simulink model "metux_controller"  (R2025b)
settings: Solver=FixedStepDiscrete  StartTime=0.0  StopTime=10  FixedStep=1/1000  RelTol=1e-3
InitFcn:
  | motor_parameters;
  | plant_parameters;
  | %load("dropLookup.mat");
  | %load("force_function.mat");
model workspace (MAT data in the model file):
  stepGain = 60
values from neighbouring files (symbols this model uses):
  enableKalmanForPositionEst = 1    [motor_parameters.m]
  enableKalmanForVelocityEst = 1    [motor_parameters.m]
  position_controller_Ts = 1e-3    (= 0.001)    [motor_parameters.m]
  velocity_controller_Ts = 1e-3    (= 0.001)    [motor_parameters.m]
libraries: subsystems x4
settings Model: TunableVars=enableKalmanForPositionEst,enableKalmanForVelocityEst,position_controller,velocity_controller,lidar_height,kalkis_target_height,Nozzle,Cmdot,attitude_controller,hwil  TunableVarsStorageClass=ExportedGlobal,ExportedGlobal,ExportedGlobal,ExportedGlobal,Auto,Auto,Auto,Auto,Auto,Auto  TunableVarsTypeQualifier=,,,,,,,,,  Creator=karadeli  LastModifiedBy=karadeli
settings OptimizationCC: DefaultParameterBehavior=Inlined  GainParamInheritBuiltInType=on  UseFloatMulNetSlope=on  StrengthReduction=on  PassReuseOutputArgsAs=Individual arguments  EfficientFloat2IntCast=on  OptimizeBlockOrder=speed  OptimizationPriority=Speed  OptimizationCustomize=off  MultiThreadedLoops=on  AutoScheduleForLoops=on  EfficientTunableParamExpr=on
settings DebuggingCC: AlgebraicLoopMsg=error  ParameterTunabilityLossMsg=error  SignalLabelMismatchMsg=warning  UnconnectedInputMsg=warning  UnconnectedOutputMsg=warning  StateNameClashWarn=warning  SFUnexpectedBacktrackingDiag=warning  SFNoUnconditionalDefaultTransitionDiag=warning  AllowAutomaticUnitConversions=off
settings HardwareCC: ProdBitPerPointer=32.0  ProdBitPerSizeT=32.0  ProdBitPerPtrDiffT=32.0  ProdLargestAtomicInteger=Long  ProdLargestAtomicFloat=Double  ProdWordSize=32.0  ProdHWDeviceType=ARM Compatible->ARM Cortex-M
settings ModelReferenceCC: ModelReferenceMinAlgLoopOccurrences=on
settings SFSimCC: MATLABDynamicMemAlloc=off
settings RTWCC: SystemTargetFile=ert.tlc  GenCodeOnly=on  PackageGeneratedCodeAndArtifacts=on  TemplateMakefile=ert_default_tmf  GenerateReport=on  BuildConfiguration=Faster Runs  LaunchReport=on  GenerateWebview=on  GenerateCodeMetricsReport=on  CheckMdlBeforeBuild=Warning  GPUComputeCapability=3.5  Description=Embedded Coder
settings CodeAppCC: ForceParamTrailComments=on  IgnoreCustomStorageClasses=off  OperatorAnnotations=on  SimulinkDataObjDesc=on  SFDataObjDesc=on  InsertBlockDesc=on  EnableCustomComments=on
settings ERTTargetCC: InlinedParameterPlacement=Hierarchical  ERTCustomFileTemplate=example_file_process.tlc  TargetLangStandard=C99 (ISO)  GenerateSampleERTMain=on  IncludeMdlTerminateFcn=off  SupportAbsoluteTime=off  SupportNonFinite=off  SupportComplex=off

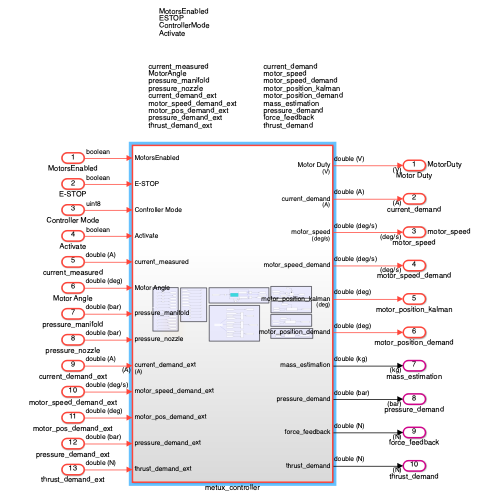
[thumbnail: Simulink's stored preview of the top-level diagram]
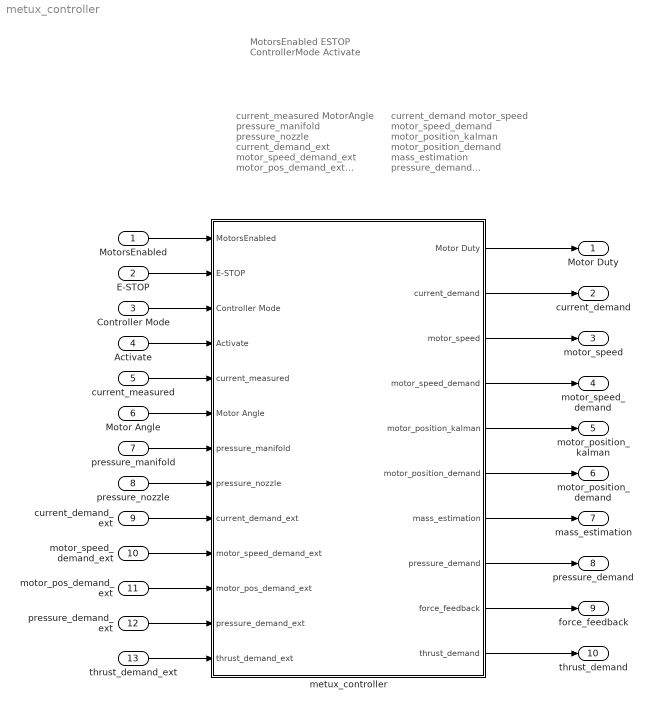
== system metux_controller ==
  note: current_demand
      | motor_speed
      | motor_speed_demand
      | motor_position_kalman
      | motor_position_demand
      | mass_estimation
      | pressure_demand
      | force_feedback
      | thrust_demand
  note: MotorsEnabled
      | ESTOP
      | ControllerMode
      | Activate
  note: current_measured
      | MotorAngle
      | pressure_manifold
      | pressure_nozzle
      | current_demand_ext
      | motor_speed_demand_ext
      | motor_pos_demand_ext
      | pressure_demand_ext
      | thrust_demand_ext
  MotorsEnabled : Inport  PortDimensions=1
  E-STOP : Inport  Port=2  PortDimensions=1
  Controller Mode : Inport  Port=3  PortDimensions=1
  Activate : Inport  Port=4  PortDimensions=1
  current_measured : Inport  Port=5  Unit=A
  Motor Angle : Inport  Port=6  Unit=deg  PortDimensions=1
  pressure_manifold : Inport  Port=7  Unit=bar
  pressure_nozzle : Inport  Port=8  Unit=bar
  current_demand_ext : Inport  Port=9
  motor_speed_demand_ext : Inport  Port=10  Unit=deg/s
  motor_pos_demand_ext : Inport  Port=11
  pressure_demand_ext : Inport  Port=12  Unit=bar
  thrust_demand_ext : Inport  Port=13  Unit=N
  metux_controller : Subsystem
  Motor Duty : Outport  SignalName=MotorDuty  Unit=V  PortDimensions=1
  current_demand : Outport  Port=2  Unit=A
  motor_speed : Outport  Port=3  SignalName=motor_speed  Unit=deg/s  PortDimensions=1
  motor_speed_demand : Outport  Port=4  Unit=deg/s  PortDimensions=1
  motor_position_kalman : Outport  Port=5
  motor_position_demand : Outport  Port=6
  mass_estimation : Outport  Port=7  Unit=kg
  pressure_demand : Outport  Port=8  Unit=bar  PortDimensions=1
  force_feedback : Outport  Port=9  Unit=N  PortDimensions=1
  thrust_demand : Outport  Port=10  Unit=N  PortDimensions=1
  wires:
  metux_controller/1(Motor Duty) -> Motor Duty/1
  pressure_manifold/1 -> metux_controller/7(pressure_manifold)
  Motor Angle/1 -> metux_controller/6(Motor Angle)
  E-STOP/1 -> metux_controller/2(E-STOP)
  Controller Mode/1 -> metux_controller/3(Controller Mode)
  Activate/1 -> metux_controller/4(Activate)
  metux_controller/3(motor_speed) -> motor_speed/1
  metux_controller/5(motor_position_kalman) -> motor_position_kalman/1
  metux_controller/4(motor_speed_demand) -> motor_speed_demand/1
  MotorsEnabled/1 -> metux_controller/1(MotorsEnabled)
  metux_controller/2(current_demand) -> current_demand/1
  metux_controller/6(motor_position_demand) -> motor_position_demand/1
  metux_controller/7(mass_estimation) -> mass_estimation/1
  metux_controller/8(pressure_demand) -> pressure_demand/1
  metux_controller/9(force_feedback) -> force_feedback/1
  metux_controller/10(thrust_demand) -> thrust_demand/1
  current_measured/1 -> metux_controller/5(current_measured)
  pressure_nozzle/1 -> metux_controller/8(pressure_nozzle)
  current_demand_ext/1 -> metux_controller/9(current_demand_ext)
  motor_speed_demand_ext/1 -> metux_controller/10(motor_speed_demand_ext)
  motor_pos_demand_ext/1 -> metux_controller/11(motor_pos_demand_ext)
  pressure_demand_ext/1 -> metux_controller/12(pressure_demand_ext)
  thrust_demand_ext/1 -> metux_controller/13(thrust_demand_ext)

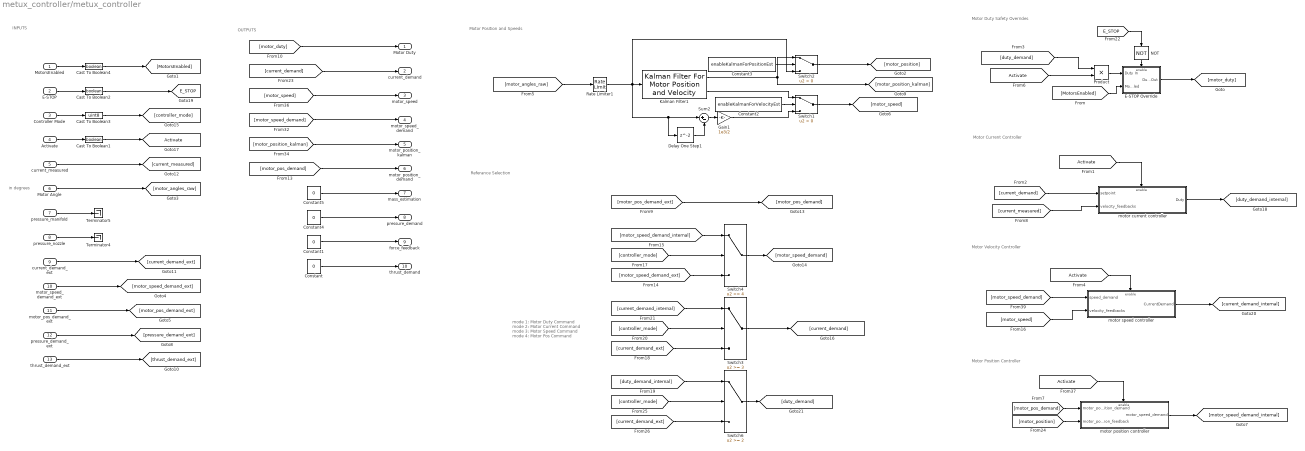
== system metux_controller/metux_controller ==
  note: Motor Current Controller
  note: Referance Selection
  note: Motor Velocity Controller
  note: Motor Duty Safety Overrides
  note: Motor Position Controller
  note: Motor Position and Speeds
  note: OUTPUTS
  note: INPUTS
  note: in degrees
  note: mode 1: Motor Duty Command
      | mode 2: Motor Current Command
      | mode 3: Motor Speed Command
      | mode 4: Motor Pos Command
  MotorsEnabled : Inport
  E-STOP : Inport  Port=2  PortDimensions=1
  Controller Mode : Inport  Port=3
  Activate : Inport  Port=4  PortDimensions=1
  current_measured : Inport  Port=5
  Motor Angle : Inport  Port=6  PortDimensions=1
  pressure_manifold : Inport  Port=7  PortDimensions=1
  pressure_nozzle : Inport  Port=8
  current_demand_ext : Inport  Port=9  Unit=A
  motor_speed_demand_ext : Inport  Port=10
  motor_pos_demand_ext : Inport  Port=11
  pressure_demand_ext : Inport  Port=12
  thrust_demand_ext : Inport  Port=13
  Cast To Boolean1 : DataTypeConversion  OutDataTypeStr=boolean  SaturateOnIntegerOverflow=off  RndMeth=Floor
  Cast To Boolean2 : DataTypeConversion  OutDataTypeStr=boolean  SaturateOnIntegerOverflow=off  RndMeth=Floor
  Cast To Boolean3 : DataTypeConversion  OutDataTypeStr=uint8  SaturateOnIntegerOverflow=off  RndMeth=Floor
  Cast To Boolean4 : DataTypeConversion  OutDataTypeStr=boolean  SaturateOnIntegerOverflow=off  RndMeth=Floor
  Constant{,1,4..5} (4 alike) : Constant  Value=0
  Constant2 : Constant  Value=enableKalmanForVelocityEst
  Constant3 : Constant  Value=enableKalmanForPositionEst
  Delay One Step1 : Delay
  E-STOP Override : Subsystem  TreatAsAtomicUnit=on
  Gain1 : Gain  Gain=1e3/2
  Kalman Filter1 : subsystems/Kalman Filter For Motor Position and Velocity  Ts=1e-3
  NOT : Logic  Operator=NOT  IconShape=distinctive  AllPortsSameDT=off  OutDataTypeStr=boolean
  Product : Product
  Rate Limiter1 : RateLimiter  RisingSlewLimit=480*360/60  FallingSlewLimit=-480*360/60  SampleTimeMode=inherited
  Sum2 : Sum  Inputs=|+-
  Switch1 : Switch  Criteria=u2 > Threshold  SaturateOnIntegerOverflow=off  InputSameDT=off
  Switch2 : Switch  Criteria=u2 > Threshold  SaturateOnIntegerOverflow=off  InputSameDT=off
  Switch3 : Switch  Threshold=3  SaturateOnIntegerOverflow=off  InputSameDT=off
  Switch4 : Switch  Threshold=4  SaturateOnIntegerOverflow=off  InputSameDT=off
  Switch6 : Switch  Threshold=2  SaturateOnIntegerOverflow=off  InputSameDT=off
  Terminator4 : Terminator
  Terminator5 : Terminator
  motor current controller : Subsystem
  motor position controller : Subsystem
  motor speed controller : Subsystem
  Motor Duty : Outport  Unit=V  PortDimensions=1
  current_demand : Outport  Port=2  Unit=A
  motor_speed : Outport  Port=3  Unit=deg/s
  motor_speed_demand : Outport  Port=4
  motor_position_kalman : Outport  Port=5  Unit=deg  PortDimensions=1
  motor_position_demand : Outport  Port=6
  mass_estimation : Outport  Port=7
  pressure_demand : Outport  Port=8
  force_feedback : Outport  Port=9
  thrust_demand : Outport  Port=10
  tag scope: Activate=global, E_STOP=global
  wires:
  E-STOP Override/1(Duty Out) -> [motor_duty]
  E-STOP/1 -> Cast To Boolean2/1
  NOT/1 -> E-STOP Override/Enable
  Controller Mode/1 -> Cast To Boolean3/1
  Activate/1 -> Cast To Boolean1/1
  motor speed controller/1(CurrentDemand) -> [current_demand_internal]
  Motor Angle/1 -> [motor_angles_raw]
  pressure_manifold/1 -> Terminator5/1
  [motor_duty] -> Motor Duty/1
  [E_STOP] -> NOT/1
  [Activate] -> motor speed controller/Enable
  [motor_speed] -> motor_speed/1
  [motor_speed] -> motor speed controller/2(velocity_feedbacks)
  [motor_position_kalman] -> motor_position_kalman/1
  [motor_speed_demand] -> motor speed controller/1(speed_demand)
  [motor_angles_raw] -> Rate Limiter1/1
  Delay One Step1/1 -> Sum2/2
  Sum2/1 -> Gain1/1
  Constant2/1 -> Switch1/2
  Gain1/1 -> Switch1/3
  Constant3/1 -> Switch2/2
  Switch2/1 -> [motor_position]
  Switch1/1 -> [motor_speed]
  [motor_position] -> motor position controller/2(motor_position_feedback)
  [Activate] -> motor position controller/Enable
  motor position controller/1(motor_speed_demand) -> [motor_speed_demand_internal]
  [motor_pos_demand] -> motor position controller/1(motor_position_demand)
  Cast To Boolean1/1 -> [Activate]
  Cast To Boolean3/1 -> [controller_mode]
  Rate Limiter1/1 -> Delay One Step1/1, Sum2/1, Kalman Filter1/1, Switch2/3
  Kalman Filter1/1 -> Switch2/1, [motor_position_kalman]
  Kalman Filter1/2 -> Switch1/1
  Product/1 -> E-STOP Override/1(Duty In)
  [motor_speed_demand] -> motor_speed_demand/1
  MotorsEnabled/1 -> Cast To Boolean4/1
  Cast To Boolean4/1 -> [MotorsEnabled]
  [MotorsEnabled] -> E-STOP Override/2(Motors Enabled)
  thrust_demand_ext/1 -> [thrust_demand_ext]
  pressure_demand_ext/1 -> [pressure_demand_ext]
  motor_pos_demand_ext/1 -> [motor_pos_demand_ext]
  motor_speed_demand_ext/1 -> [motor_speed_demand_ext]
  pressure_nozzle/1 -> Terminator4/1
  current_demand_ext/1 -> [current_demand_ext]
  current_measured/1 -> [current_measured]
  Constant/1 -> thrust_demand/1
  Constant1/1 -> force_feedback/1
  Constant4/1 -> pressure_demand/1
  Constant5/1 -> mass_estimation/1
  [motor_pos_demand] -> motor_position_demand/1
  [motor_pos_demand_ext] -> [motor_pos_demand]
  [controller_mode] -> Switch4/2
  [motor_speed_demand_internal] -> Switch4/1
  [motor_speed_demand_ext] -> Switch4/3
  Switch4/1 -> [motor_speed_demand]
  [controller_mode] -> Switch3/2
  [Activate] -> motor current controller/Enable
  motor current controller/1(Duty) -> [duty_demand_internal]
  [current_demand] -> motor current controller/1(setpoint)
  [current_measured] -> motor current controller/2(velocity_feedbacks)
  [duty_demand_internal] -> Switch6/1
  [controller_mode] -> Switch6/2
  [current_demand_ext] -> Switch6/3
  Switch6/1 -> [duty_demand]
  [duty_demand] -> Product/1
  [Activate] -> Product/2
  [current_demand] -> current_demand/1
  [current_demand_ext] -> Switch3/3
  [current_demand_internal] -> Switch3/1
  Switch3/1 -> [current_demand]
  Cast To Boolean2/1 -> [E_STOP]

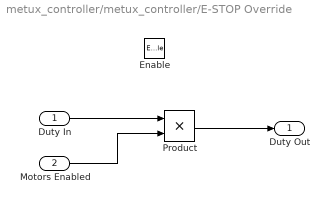
== system metux_controller/metux_controller/E-STOP Override ==
  Duty In : Inport  Unit=V  PortDimensions=1
  Motors Enabled : Inport  Port=2
  Enable : EnablePort  StatesWhenEnabling=reset
  Product : Product
  Duty Out : Outport  Unit=V  PortDimensions=1  OutputWhenDisabled=reset  InitialOutput=[0]
  wires:
  Product/1 -> Duty Out/1
  Duty In/1 -> Product/1
  Motors Enabled/1 -> Product/2

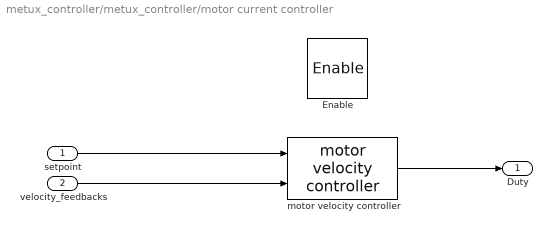
== system metux_controller/metux_controller/motor current controller ==
  setpoint : Inport  Unit=A  SampleTime=velocity_controller_Ts
  velocity_feedbacks : Inport  Port=2  Unit=A  SampleTime=velocity_controller_Ts
  Enable : EnablePort
  motor velocity controller : subsystems/motor velocity controller  SystemSampleTime=-1  VariantActivationTime=update diagram  EmptyChoice=off  PassThrough=off  PassThroughVariantControl=(default)  EmptyChoiceVariantControl=(default)  AllowFlexibleInterface=on  Latency=0  AutoFrameSizeCalculation=off
  Duty : Outport  Unit=V  PortDimensions=1  SampleTime=velocity_controller_Ts  OutputWhenDisabled=reset  InitialOutput=0
  wires:
  velocity_feedbacks/1 -> motor velocity controller/2
  motor velocity controller/1 -> Duty/1
  setpoint/1 -> motor velocity controller/1

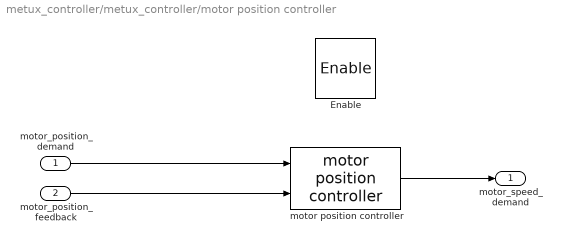
== system metux_controller/metux_controller/motor position controller ==
  motor_position_demand : Inport  Unit=deg  PortDimensions=1  SampleTime=position_controller_Ts
  motor_position_feedback : Inport  Port=2  SampleTime=position_controller_Ts
  Enable : EnablePort
  motor position controller : subsystems/motor position controller  SystemSampleTime=-1  VariantActivationTime=update diagram  EmptyChoice=off  PassThrough=off  PassThroughVariantControl=(default)  EmptyChoiceVariantControl=(default)  AllowFlexibleInterface=on  Latency=0  AutoFrameSizeCalculation=off
  motor_speed_demand : Outport  Unit=deg/s  PortDimensions=1  SampleTime=position_controller_Ts  OutputWhenDisabled=reset  InitialOutput=0
  wires:
  motor_position_feedback/1 -> motor position controller/2
  motor position controller/1 -> motor_speed_demand/1
  motor_position_demand/1 -> motor position controller/1

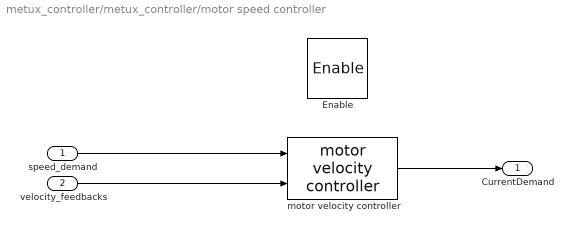
== system metux_controller/metux_controller/motor speed controller ==
  speed_demand : Inport  Unit=deg/s  SampleTime=velocity_controller_Ts
  velocity_feedbacks : Inport  Port=2  Unit=deg/s  SampleTime=velocity_controller_Ts
  Enable : EnablePort
  motor velocity controller : subsystems/motor velocity controller  SystemSampleTime=-1  VariantActivationTime=update diagram  EmptyChoice=off  PassThrough=off  PassThroughVariantControl=(default)  EmptyChoiceVariantControl=(default)  AllowFlexibleInterface=on  Latency=0  AutoFrameSizeCalculation=off
  CurrentDemand : Outport  Unit=A  PortDimensions=1  SampleTime=velocity_controller_Ts  OutputWhenDisabled=reset  InitialOutput=0
  wires:
  speed_demand/1 -> motor velocity controller/1
  motor velocity controller/1 -> CurrentDemand/1
  velocity_feedbacks/1 -> motor velocity controller/2
